simulink model "PlanarRobot5link"  (R2022b)
settings: Solver=VariableStepAuto  StartTime=0.0  StopTime=30  RelTol=1e-3
values from neighbouring files (symbols this model uses):
  I = [1; 1; 1; 0.5; 0.5]*0.2    [RobDyn4link.m]
  l = [1; 1; 1; 1; 2]*0.2    [RobDyn4link.m]
  lc = l./2    [RobDyn4link.m]
  m = [1; 1; 1; 0.3; 0.3]*1    [RobDyn4link.m]
  q0 = [pi/2; -pi/4; -1*pi/6;-pi/12;0;]    [RobDyn4link.m]
  theta_max = [0.915*pi; 0.915*pi; 0.915*pi; 0.915*pi; 0.915*pi;]    [RobDyn4link.m]
  theta_min = [-0.915*pi; -0.915*pi; -0.915*pi; -0.915*pi; -0.915*pi;]    [RobDyn4link.m]
libraries: slpidlib x1
(part 2 of 3)

== matlab function PlanarRobot5link/Subsystem1/MATLAB Function ==
  data: theta input; C output; dtheta input; m input; l input; lc input
function C = fcn(theta,dtheta,m,l,lc)
theta1 = theta(1); theta2 = theta(2); theta3 = theta(3); theta4 = theta(4); theta5 = theta(5);
dtheta1 = dtheta(1); dtheta2 = dtheta(2); dtheta3 = dtheta(3); dtheta4 = dtheta(4); dtheta5 = dtheta(5);
% I1 = I(1); I2 = I(2); I3 = I(3); I4 = I(4); I5 = I(5);
m1 = m(1); m2 = m(2); m3 = m(3); m4 = m(4); m5 = m(5);
l1 = l(1); l2 = l(2); l3 = l(3); l4 = l(4); l5 = l(5);
lc1 = lc(1); lc2 = lc(2); lc3 = lc(3); lc4 = lc(4); lc5 = lc(5);

 
C =[- dtheta2*l1*l4*m5*sin(theta2 + theta3 + theta4) - dtheta3*l1*l4*m5*sin(theta2 + theta3 + theta4) - dtheta4*l1*l4*m5*sin(theta2 + theta3 + theta4) - dtheta2*l1*lc4*m4*sin(theta2 + theta3 + theta4) - dtheta3*l1*lc4*m4*sin(theta2 + theta3 + theta4) - dtheta4*l1*lc4*m4*sin(theta2 + theta3 + theta4) - dtheta3*l2*lc5*m5*sin(theta3 + theta4 + theta5) - dtheta4*l2*lc5*m5*sin(theta3 + theta4 + theta5) - dtheta5*l2*lc5*m5*sin(theta3 + theta4 + theta5) - dtheta2*l1*lc5*m5*sin(theta2 + theta3 + theta4 + theta5) - dtheta3*l1*lc5*m5*sin(theta2 + theta3 + theta4 + theta5) - dtheta4*l1*lc5*m5*sin(theta2 + theta3 + theta4 + theta5) - dtheta5*l1*lc5*m5*sin(theta2 + theta3 + theta4 + theta5) - dtheta2*l1*l3*m4*sin(theta2 + theta3) - dtheta2*l1*l3*m5*sin(theta2 + theta3) - dtheta3*l1*l3*m4*sin(theta2 + theta3) - dtheta3*l1*l3*m5*sin(theta2 + theta3) - dtheta3*l2*l4*m5*sin(theta3 + theta4) - dtheta4*l2*l4*m5*sin(theta3 + theta4) - dtheta2*l1*lc3*m3*sin(theta2 + theta3) - dtheta3*l1*lc3*m3*sin(theta2 + theta3) - dtheta3*l2*lc4*m4*sin(theta3 + theta4) - dtheta4*l2*lc4*m4*sin(theta3 + theta4) - dtheta4*l3*lc5*m5*sin(theta4 + theta5) - dtheta5*l3*lc5*m5*sin(theta4 + theta5) - dtheta2*l1*l2*m3*sin(theta2) - dtheta2*l1*l2*m4*sin(theta2) - dtheta2*l1*l2*m5*sin(theta2) - dtheta3*l2*l3*m4*sin(theta3) - dtheta3*l2*l3*m5*sin(theta3) - dtheta4*l3*l4*m5*sin(theta4) - dtheta2*l1*lc2*m2*sin(theta2) - dtheta3*l2*lc3*m3*sin(theta3) - dtheta4*l3*lc4*m4*sin(theta4) - dtheta5*l4*lc5*m5*sin(theta5), - dtheta1*l1*l4*m5*sin(theta2 + theta3 + theta4) - dtheta2*l1*l4*m5*sin(theta2 + theta3 + theta4) - dtheta3*l1*l4*m5*sin(theta2 + theta3 + theta4) - dtheta4*l1*l4*m5*sin(theta2 + theta3 + theta4) - dtheta1*l1*lc4*m4*sin(theta2 + theta3 + theta4) - dtheta2*l1*lc4*m4*sin(theta2 + theta3 + theta4) - dtheta3*l1*lc4*m4*sin(theta2 + theta3 + theta4) - dtheta4*l1*lc4*m4*sin(theta2 + theta3 + theta4) - dtheta3*l2*lc5*m5*sin(theta3 + theta4 + theta5) - dtheta4*l2*lc5*m5*sin(theta3 + theta4 + theta5) - dtheta5*l2*lc5*m5*sin(theta3 + theta4 + theta5) - dtheta1*l1*lc5*m5*sin(theta2 + theta3 + theta4 + theta5) - dtheta2*l1*lc5*m5*sin(theta2 + theta3 + theta4 + theta5) - dtheta3*l1*lc5*m5*sin(theta2 + theta3 + theta4 + theta5) - dtheta4*l1*lc5*m5*sin(theta2 + theta3 + theta4 + theta5) - dtheta5*l1*lc5*m5*sin(theta2 + theta3 + theta4 + theta5) - dtheta1*l1*l3*m4*sin(theta2 + theta3) - dtheta1*l1*l3*m5*sin(theta2 + theta3) - dtheta2*l1*l3*m4*sin(theta2 + theta3) - dtheta2*l1*l3*m5*sin(theta2 + theta3) - dtheta3*l1*l3*m4*sin(theta2 + theta3) - dtheta3*l1*l3*m5*sin(theta2 + theta3) - dtheta3*l2*l4*m5*sin(theta3 + theta4) - dtheta4*l2*l4*m5*sin(theta3 + theta4) - dtheta1*l1*lc3*m3*sin(theta2 + theta3) - dtheta2*l1*lc3*m3*sin(theta2 + theta3) - dtheta3*l1*lc3*m3*sin(theta2 + theta3) - dtheta3*l2*lc4*m4*sin(theta3 + theta4) - dtheta4*l2*lc4*m4*sin(theta3 + theta4) - dtheta4*l3*lc5*m5*sin(theta4 + theta5) - dtheta5*l3*lc5*m5*sin(theta4 + theta5) - dtheta1*l1*l2*m3*sin(theta2) - dtheta1*l1*l2*m4*sin(theta2) - dtheta2*l1*l2*m3*sin(theta2) - dtheta1*l1*l2*m5*sin(theta2) - dtheta2*l1*l2*m4*sin(theta2) - dtheta2*l1*l2*m5*sin(theta2) - dtheta3*l2*l3*m4*sin(theta3) - dtheta3*l2*l3*m5*sin(theta3) - dtheta4*l3*l4*m5*sin(theta4) - dtheta1*l1*lc2*m2*sin(theta2) - dtheta2*l1*lc2*m2*sin(theta2) - dtheta3*l2*lc3*m3*sin(theta3) - dtheta4*l3*lc4*m4*sin(theta4) - dtheta5*l4*lc5*m5*sin(theta5), - dtheta1*l1*l4*m5*sin(theta2 + theta3 + theta4) - dtheta2*l1*l4*m5*sin(theta2 + theta3 + theta4) - dtheta3*l1*l4*m5*sin(theta2 + theta3 + theta4) - dtheta4*l1*l4*m5*sin(theta2 + theta3 + theta4) - dtheta1*l1*lc4*m4*sin(theta2 + theta3 + theta4) - dtheta2*l1*lc4*m4*sin(theta2 + theta3 + theta4) - dtheta3*l1*lc4*m4*sin(theta2 + theta3 + theta4) - dtheta4*l1*lc4*m4*sin(theta2 + theta3 + theta4) - dtheta1*l2*lc5*m5*sin(theta3 + theta4 + theta5) - dtheta2*l2*lc5*m5*sin(theta3 + theta4 + theta5) - dtheta3*l2*lc5*m5*sin(theta3 + theta4 + theta5) - dtheta4*l2*lc5*m5*sin(theta3 + theta4 + theta5) - dtheta5*l2*lc5*m5*sin(theta3 + theta4 + theta5) - dtheta1*l1*lc5*m5*sin(theta2 + theta3 + theta4 + theta5) - dtheta2*l1*lc5*m5*sin(theta2 + theta3 + theta4 + theta5) - dtheta3*l1*lc5*m5*sin(theta2 + theta3 + theta4 + theta5) - dtheta4*l1*lc5*m5*sin(theta2 + theta3 + theta4 + theta5) - dtheta5*l1*lc5*m5*sin(theta2 + theta3 + theta4 + theta5) - dtheta1*l1*l3*m4*sin(theta2 + theta3) - dtheta1*l1*l3*m5*sin(theta2 + theta3) - dtheta2*l1*l3*m4*sin(theta2 + theta3) - dtheta2*l1*l3*m5*sin(theta2 + theta3) - dtheta3*l1*l3*m4*sin(theta2 + theta3) - dtheta3*l1*l3*m5*sin(theta2 + theta3) - dtheta1*l2*l4*m5*sin(theta3 + theta4) - dtheta2*l2*l4*m5*sin(theta3 + theta4) - dtheta3*l2*l4*m5*sin(theta3 + theta4) - dtheta4*l2*l4*m5*sin(theta3 + theta4) - dtheta1*l1*lc3*m3*sin(theta2 + theta3) - dtheta2*l1*lc3*m3*sin(theta2 + theta3) - dtheta3*l1*lc3*m3*sin(theta2 + theta3) - dtheta1*l2*lc4*m4*sin(theta3 + theta4) - dtheta2*l2*lc4*m4*sin(theta3 + theta4) - dtheta3*l2*lc4*m4*sin(theta3 + theta4) - dtheta4*l2*lc4*m4*sin(theta3 + theta4) - dtheta4*l3*lc5*m5*sin(theta4 + theta5) - dtheta5*l3*lc5*m5*sin(theta4 + theta5) - dtheta1*l2*l3*m4*sin(theta3) - dtheta1*l2*l3*m5*sin(theta3) - dtheta2*l2*l3*m4*sin(theta3) - dtheta2*l2*l3*m5*sin(theta3) - dtheta3*l2*l3*m4*sin(theta3) - dtheta3*l2*l3*m5*sin(theta3) - dtheta4*l3*l4*m5*sin(theta4) - dtheta1*l2*lc3*m3*sin(theta3) - dtheta2*l2*lc3*m3*sin(theta3) - dtheta3*l2*lc3*m3*sin(theta3) - dtheta4*l3*lc4*m4*sin(theta4) - dtheta5*l4*lc5*m5*sin(theta5), - dtheta1*l1*l4*m5*sin(theta2 + theta3 + theta4) - dtheta2*l1*l4*m5*sin(theta2 + theta3 + theta4) - dtheta3*l1*l4*m5*sin(theta2 + theta3 + theta4) - dtheta4*l1*l4*m5*sin(theta2 + theta3 + theta4) - dtheta1*l1*lc4*m4*sin(theta2 + theta3 + theta4) - dtheta2*l1*lc4*m4*sin(theta2 + theta3 + theta4) - dtheta3*l1*lc4*m4*sin(theta2 + theta3 + theta4) - dtheta4*l1*lc4*m4*sin(theta2 + theta3 + theta4) - dtheta1*l2*lc5*m5*sin(theta3 + theta4 + theta5) - dtheta2*l2*lc5*m5*sin(theta3 + theta4 + theta5) - dtheta3*l2*lc5*m5*sin(theta3 + theta4 + theta5) - dtheta4*l2*lc5*m5*sin(theta3 + theta4 + theta5) - dtheta5*l2*lc5*m5*sin(theta3 + theta4 + theta5) - dtheta1*l1*lc5*m5*sin(theta2 + theta3 + theta4 + theta5) - dtheta2*l1*lc5*m5*sin(theta2 + theta3 + theta4 + theta5) - dtheta3*l1*lc5*m5*sin(theta2 + theta3 + theta4 + theta5) - dtheta4*l1*lc5*m5*sin(theta2 + theta3 + theta4 + theta5) - dtheta5*l1*lc5*m5*sin(theta2 + theta3 + theta4 + theta5) - dtheta1*l2*l4*m5*sin(theta3 + theta4) - dtheta2*l2*l4*m5*sin(theta3 + theta4) - dtheta3*l2*l4*m5*sin(theta3 + theta4) - dtheta4*l2*l4*m5*sin(theta3 + theta4) - dtheta1*l2*lc4*m4*sin(theta3 + theta4) - dtheta2*l2*lc4*m4*sin(theta3 + theta4) - dtheta3*l2*lc4*m4*sin(theta3 + theta4) - dtheta4*l2*lc4*m4*sin(theta3 + theta4) - dtheta1*l3*lc5*m5*sin(theta4 + theta5) - dtheta2*l3*lc5*m5*sin(theta4 + theta5) - dtheta3*l3*lc5*m5*sin(theta4 + theta5) - dtheta4*l3*lc5*m5*sin(theta4 + theta5) - dtheta5*l3*lc5*m5*sin(theta4 + theta5) - dtheta1*l3*l4*m5*sin(theta4) - dtheta2*l3*l4*m5*sin(theta4) - dtheta3*l3*l4*m5*sin(theta4) - dtheta4*l3*l4*m5*sin(theta4) - dtheta1*l3*lc4*m4*sin(theta4) - dtheta2*l3*lc4*m4*sin(theta4) - dtheta3*l3*lc4*m4*sin(theta4) - dtheta4*l3*lc4*m4*sin(theta4) - dtheta5*l4*lc5*m5*sin(theta5), -lc5*m5*(l1*sin(theta2 + theta3 + theta4 + theta5) + l3*sin(theta4 + theta5) + l4*sin(theta5) + l2*sin(theta3 + theta4 + theta5))*(dtheta1 + dtheta2 + dtheta3 + dtheta4 + dtheta5);
                                                                                                                                                                                                                                                                                                                                                                                                                                                                                                                  dtheta1*l1*l4*m5*sin(theta2 + theta3 + theta4) + dtheta1*l1*lc4*m4*sin(theta2 + theta3 + theta4) - dtheta3*l2*lc5*m5*sin(theta3 + theta4 + theta5) - dtheta4*l2*lc5*m5*sin(theta3 + theta4 + theta5) - dtheta5*l2*lc5*m5*sin(theta3 + theta4 + theta5) + dtheta1*l1*lc5*m5*sin(theta2 + theta3 + theta4 + theta5) + dtheta1*l1*l3*m4*sin(theta2 + theta3) + dtheta1*l1*l3*m5*sin(theta2 + theta3) - dtheta3*l2*l4*m5*sin(theta3 + theta4) - dtheta4*l2*l4*m5*sin(theta3 + theta4) + dtheta1*l1*lc3*m3*sin(theta2 + theta3) - dtheta3*l2*lc4*m4*sin(theta3 + theta4) - dtheta4*l2*lc4*m4*sin(theta3 + theta4) - dtheta4*l3*lc5*m5*sin(theta4 + theta5) - dtheta5*l3*lc5*m5*sin(theta4 + theta5) + dtheta1*l1*l2*m3*sin(theta2) + dtheta1*l1*l2*m4*sin(theta2) + dtheta1*l1*l2*m5*sin(theta2) - dtheta3*l2*l3*m4*sin(theta3) - dtheta3*l2*l3*m5*sin(theta3) - dtheta4*l3*l4*m5*sin(theta4) + dtheta1*l1*lc2*m2*sin(theta2) - dtheta3*l2*lc3*m3*sin(theta3) - dtheta4*l3*lc4*m4*sin(theta4) - dtheta5*l4*lc5*m5*sin(theta5),                                                                                                                                                                                                                                                                                                                                                                                                                                                                                                                                                                                                                                                                                                                                                                                                                                                                                                                                                                                                                                                                                                                                                                                                                                                                                                                                                                                                                                                                                - dtheta4*(l2*l4*m5*sin(theta3 + theta4) + l2*lc4*m4*sin(theta3 + theta4) + l3*lc5*m5*sin(theta4 + theta5) + l3*l4*m5*sin(theta4) + l3*lc4*m4*sin(theta4) + l2*lc5*m5*sin(theta3 + theta4 + theta5)) - dtheta3*l2*(l3*m4*sin(theta3) + l3*m5*sin(theta3) + lc3*m3*sin(theta3) + lc5*m5*sin(theta3 + theta4 + theta5) + l4*m5*sin(theta3 + theta4) + lc4*m4*sin(theta3 + theta4)) - dtheta5*lc5*m5*(l3*sin(theta4 + theta5) + l4*sin(theta5) + l2*sin(theta3 + theta4 + theta5)),                                                                                                                                                                                                                                                                                                                                                                                                                                                                                                                                                                                                                                                                                                                                                                                                                                                                                                                                                                                                                                                                                               - dtheta1*l2*lc5*m5*sin(theta3 + theta4 + theta5) - dtheta2*l2*lc5*m5*sin(theta3 + theta4 + theta5) - dtheta3*l2*lc5*m5*sin(theta3 + theta4 + theta5) - dtheta4*l2*lc5*m5*sin(theta3 + theta4 + theta5) - dtheta5*l2*lc5*m5*sin(theta3 + theta4 + theta5) - dtheta1*l2*l4*m5*sin(theta3 + theta4) - dtheta2*l2*l4*m5*sin(theta3 + theta4) - dtheta3*l2*l4*m5*sin(theta3 + theta4) - dtheta4*l2*l4*m5*sin(theta3 + theta4) - dtheta1*l2*lc4*m4*sin(theta3 + theta4) - dtheta2*l2*lc4*m4*sin(theta3 + theta4) - dtheta3*l2*lc4*m4*sin(theta3 + theta4) - dtheta4*l2*lc4*m4*sin(theta3 + theta4) - dtheta4*l3*lc5*m5*sin(theta4 + theta5) - dtheta5*l3*lc5*m5*sin(theta4 + theta5) - dtheta1*l2*l3*m4*sin(theta3) - dtheta1*l2*l3*m5*sin(theta3) - dtheta2*l2*l3*m4*sin(theta3) - dtheta2*l2*l3*m5*sin(theta3) - dtheta3*l2*l3*m4*sin(theta3) - dtheta3*l2*l3*m5*sin(theta3) - dtheta4*l3*l4*m5*sin(theta4) - dtheta1*l2*lc3*m3*sin(theta3) - dtheta2*l2*lc3*m3*sin(theta3) - dtheta3*l2*lc3*m3*sin(theta3) - dtheta4*l3*lc4*m4*sin(theta4) - dtheta5*l4*lc5*m5*sin(theta5),                                                                                                                                                                                                                                                                                                                                                                                                                                                                                                                                                                                                                                                                                                                    - dtheta1*l2*lc5*m5*sin(theta3 + theta4 + theta5) - dtheta2*l2*lc5*m5*sin(theta3 + theta4 + theta5) - dtheta3*l2*lc5*m5*sin(theta3 + theta4 + theta5) - dtheta4*l2*lc5*m5*sin(theta3 + theta4 + theta5) - dtheta5*l2*lc5*m5*sin(theta3 + theta4 + theta5) - dtheta1*l2*l4*m5*sin(theta3 + theta4) - dtheta2*l2*l4*m5*sin(theta3 + theta4) - dtheta3*l2*l4*m5*sin(theta3 + theta4) - dtheta4*l2*l4*m5*sin(theta3 + theta4) - dtheta1*l2*lc4*m4*sin(theta3 + theta4) - dtheta2*l2*lc4*m4*sin(theta3 + theta4) - dtheta3*l2*lc4*m4*sin(theta3 + theta4) - dtheta4*l2*lc4*m4*sin(theta3 + theta4) - dtheta1*l3*lc5*m5*sin(theta4 + theta5) - dtheta2*l3*lc5*m5*sin(theta4 + theta5) - dtheta3*l3*lc5*m5*sin(theta4 + theta5) - dtheta4*l3*lc5*m5*sin(theta4 + theta5) - dtheta5*l3*lc5*m5*sin(theta4 + theta5) - dtheta1*l3*l4*m5*sin(theta4) - dtheta2*l3*l4*m5*sin(theta4) - dtheta3*l3*l4*m5*sin(theta4) - dtheta4*l3*l4*m5*sin(theta4) - dtheta1*l3*lc4*m4*sin(theta4) - dtheta2*l3*lc4*m4*sin(theta4) - dtheta3*l3*lc4*m4*sin(theta4) - dtheta4*l3*lc4*m4*sin(theta4) - dtheta5*l4*lc5*m5*sin(theta5),                                             -lc5*m5*(l3*sin(theta4 + theta5) + l4*sin(theta5) + l2*sin(theta3 + theta4 + theta5))*(dtheta1 + dtheta2 + dtheta3 + dtheta4 + dtheta5);
                                                                                                                                                                                                                                                                                                                                                                                                                                                                                                                                                                                                   dtheta1*l1*l4*m5*sin(theta2 + theta3 + theta4) + dtheta1*l1*lc4*m4*sin(theta2 + theta3 + theta4) + dtheta1*l2*lc5*m5*sin(theta3 + theta4 + theta5) + dtheta2*l2*lc5*m5*sin(theta3 + theta4 + theta5) + dtheta1*l1*lc5*m5*sin(theta2 + theta3 + theta4 + theta5) + dtheta1*l1*l3*m4*sin(theta2 + theta3) + dtheta1*l1*l3*m5*sin(theta2 + theta3) + dtheta1*l2*l4*m5*sin(theta3 + theta4) + dtheta2*l2*l4*m5*sin(theta3 + theta4) + dtheta1*l1*lc3*m3*sin(theta2 + theta3) + dtheta1*l2*lc4*m4*sin(theta3 + theta4) + dtheta2*l2*lc4*m4*sin(theta3 + theta4) - dtheta4*l3*lc5*m5*sin(theta4 + theta5) - dtheta5*l3*lc5*m5*sin(theta4 + theta5) + dtheta1*l2*l3*m4*sin(theta3) + dtheta1*l2*l3*m5*sin(theta3) + dtheta2*l2*l3*m4*sin(theta3) + dtheta2*l2*l3*m5*sin(theta3) - dtheta4*l3*l4*m5*sin(theta4) + dtheta1*l2*lc3*m3*sin(theta3) + dtheta2*l2*lc3*m3*sin(theta3) - dtheta4*l3*lc4*m4*sin(theta4) - dtheta5*l4*lc5*m5*sin(theta5),                                                                                                                                                                                                                                                                                                                                                                                                                                                                                                                                                                                                                                                                                                                                                                                                                                                                                                                                                                                                                                                                                                                                                                                                                                                                                                                                                                                                               dtheta1*(l2*l4*m5*sin(theta3 + theta4) + l2*lc4*m4*sin(theta3 + theta4) + l2*l3*m4*sin(theta3) + l2*l3*m5*sin(theta3) + l2*lc3*m3*sin(theta3) + l2*lc5*m5*sin(theta3 + theta4 + theta5)) - dtheta5*(l3*lc5*m5*sin(theta4 + theta5) + l4*lc5*m5*sin(theta5)) + dtheta2*(l2*l4*m5*sin(theta3 + theta4) + l2*lc4*m4*sin(theta3 + theta4) + l2*l3*m4*sin(theta3) + l2*l3*m5*sin(theta3) + l2*lc3*m3*sin(theta3) + l2*lc5*m5*sin(theta3 + theta4 + theta5)) - dtheta4*(l3*lc5*m5*sin(theta4 + theta5) + l3*l4*m5*sin(theta4) + l3*lc4*m4*sin(theta4)),                                                                                                                                                                                                                                                                                                                                                                                                                                                                                                                                                                                                                                                                                                                                                                                                                                                                                                                                                                                                                                                                                                                                                                                                                                                                                                                                                                                                                                                                                                                                                                                                                                                                                                                                                                                                                                                                                                                                                                                                           - dtheta5*(l3*lc5*m5*sin(theta4 + theta5) + l4*lc5*m5*sin(theta5)) - dtheta4*(l3*lc5*m5*sin(theta4 + theta5) + l3*l4*m5*sin(theta4) + l3*lc4*m4*sin(theta4)),                                                                                                                                                                                                                                                                                                                                                                                                                                                                                                                                                                                                                                                                                                                                                                                                                                                                                                                                                                                                                                                                                                                                                                                                                                                                                                                                                                                                               - dtheta1*l3*(l4*m5*sin(theta4) + lc4*m4*sin(theta4) + lc5*m5*sin(theta4 + theta5)) - dtheta2*l3*(l4*m5*sin(theta4) + lc4*m4*sin(theta4) + lc5*m5*sin(theta4 + theta5)) - dtheta3*l3*(l4*m5*sin(theta4) + lc4*m4*sin(theta4) + lc5*m5*sin(theta4 + theta5)) - dtheta4*l3*(l4*m5*sin(theta4) + lc4*m4*sin(theta4) + lc5*m5*sin(theta4 + theta5)) - dtheta5*lc5*m5*(l3*sin(theta4 + theta5) + l4*sin(theta5)),                                                                                -lc5*m5*(l3*sin(theta4 + theta5) + l4*sin(theta5))*(dtheta1 + dtheta2 + dtheta3 + dtheta4 + dtheta5);
                                                                                                                                                                                                                                                                                                                                                                                                                                                                                                                                                                                                                                                                                                                                                 dtheta1*l1*l4*m5*sin(theta2 + theta3 + theta4) + dtheta1*l1*lc4*m4*sin(theta2 + theta3 + theta4) + dtheta1*l2*lc5*m5*sin(theta3 + theta4 + theta5) + dtheta2*l2*lc5*m5*sin(theta3 + theta4 + theta5) + dtheta1*l1*lc5*m5*sin(theta2 + theta3 + theta4 + theta5) + dtheta1*l2*l4*m5*sin(theta3 + theta4) + dtheta2*l2*l4*m5*sin(theta3 + theta4) + dtheta1*l2*lc4*m4*sin(theta3 + theta4) + dtheta2*l2*lc4*m4*sin(theta3 + theta4) + dtheta1*l3*lc5*m5*sin(theta4 + theta5) + dtheta2*l3*lc5*m5*sin(theta4 + theta5) + dtheta3*l3*lc5*m5*sin(theta4 + theta5) + dtheta1*l3*l4*m5*sin(theta4) + dtheta2*l3*l4*m5*sin(theta4) + dtheta3*l3*l4*m5*sin(theta4) + dtheta1*l3*lc4*m4*sin(theta4) + dtheta2*l3*lc4*m4*sin(theta4) + dtheta3*l3*lc4*m4*sin(theta4) - dtheta5*l4*lc5*m5*sin(theta5),                                                                                                                                                                                                                                                                                                                                                                                                                                                                                                                                                                                                                                                                                                                                                                                                                                                                                                                                                                                                                                                                                                                                                                                                                                                                                                                                    dtheta1*l2*lc5*m5*sin(theta3 + theta4 + theta5) + dtheta2*l2*lc5*m5*sin(theta3 + theta4 + theta5) + dtheta1*l2*l4*m5*sin(theta3 + theta4) + dtheta2*l2*l4*m5*sin(theta3 + theta4) + dtheta1*l2*lc4*m4*sin(theta3 + theta4) + dtheta2*l2*lc4*m4*sin(theta3 + theta4) + dtheta1*l3*lc5*m5*sin(theta4 + theta5) + dtheta2*l3*lc5*m5*sin(theta4 + theta5) + dtheta3*l3*lc5*m5*sin(theta4 + theta5) + dtheta1*l3*l4*m5*sin(theta4) + dtheta2*l3*l4*m5*sin(theta4) + dtheta3*l3*l4*m5*sin(theta4) + dtheta1*l3*lc4*m4*sin(theta4) + dtheta2*l3*lc4*m4*sin(theta4) + dtheta3*l3*lc4*m4*sin(theta4) - dtheta5*l4*lc5*m5*sin(theta5),                                                                                                                                                                                                                                                                                                                                                                                                                                                                                                                                                                                                                                                                                                                                                                                                                                                                                                                                                                                                                                                                                                                                                                                                                                                                                                                                                                                                                                                                                                                                                                                                                                                                                                                                                                                                                                                                              dtheta1*l3*(l4*m5*sin(theta4) + lc4*m4*sin(theta4) + lc5*m5*sin(theta4 + theta5)) + dtheta2*l3*(l4*m5*sin(theta4) + lc4*m4*sin(theta4) + lc5*m5*sin(theta4 + theta5)) + dtheta3*l3*(l4*m5*sin(theta4) + lc4*m4*sin(theta4) + lc5*m5*sin(theta4 + theta5)) - dtheta5*l4*lc5*m5*sin(theta5),                                                                                                                                                                                                                                                                                                                                                                                                                                                                                                                                                                                                                                                                                                                                                                                                                                                                                                                                                                                                                                                                                                                                                                                                                                                                                                                                                                                                                                                                                                                                                                                                                                                                                                                                                                                            -dtheta5*l4*lc5*m5*sin(theta5),                                                                                                            -l4*lc5*m5*sin(theta5)*(dtheta1 + dtheta2 + dtheta3 + dtheta4 + dtheta5);
                                                                                                                                                                                                                                                                                                                                                                                                                                                                                                                                                                                                                                                                                                                                                                                                                                                                                                                                                                                                                                                                                                                                                                                lc5*m5*(dtheta1*l4*sin(theta5) + dtheta2*l4*sin(theta5) + dtheta3*l4*sin(theta5) + dtheta4*l4*sin(theta5) + dtheta1*l2*sin(theta3 + theta4 + theta5) + dtheta2*l2*sin(theta3 + theta4 + theta5) + dtheta1*l1*sin(theta2 + theta3 + theta4 + theta5) + dtheta1*l3*sin(theta4 + theta5) + dtheta2*l3*sin(theta4 + theta5) + dtheta3*l3*sin(theta4 + theta5)),                                                                                                                                                                                                                                                                                                                                                                                                                                                                                                                                                                                                                                                                                                                                                                                                                                                                                                                                                                                                                                                                                                                                                                                                                                                                                                                                                                                                                                                                                                                                                                                                                                                         lc5*m5*(dtheta1*l4*sin(theta5) + dtheta2*l4*sin(theta5) + dtheta3*l4*sin(theta5) + dtheta4*l4*sin(theta5) + dtheta1*l2*sin(theta3 + theta4 + theta5) + dtheta2*l2*sin(theta3 + theta4 + theta5) + dtheta1*l3*sin(theta4 + theta5) + dtheta2*l3*sin(theta4 + theta5) + dtheta3*l3*sin(theta4 + theta5)),                                                                                                                                                                                                                                                                                                                                                                                                                                                                                                                                                                                                                                                                                                                                                                                                                                                                                                                                                                                                                                                                                                                                                                                                                                                                                                                                                                                                                                                                                                                                                                                                                                                                                                                                                                                                                                                                                                                                                       lc5*m5*(dtheta1*l4*sin(theta5) + dtheta2*l4*sin(theta5) + dtheta3*l4*sin(theta5) + dtheta4*l4*sin(theta5) + dtheta1*l3*sin(theta4 + theta5) + dtheta2*l3*sin(theta4 + theta5) + dtheta3*l3*sin(theta4 + theta5)),                                                                                                                                                                                                                                                                                                                                                                                                                                                                                                                                                                                                                                                                                                                                                                                                                                                                                                                                                                                                                                                                                                                                                                                                                                                                                                                                                                                                                                                                                                                                                                                                                                                                                                                                                             l4*lc5*m5*sin(theta5)*(dtheta1 + dtheta2 + dtheta3 + dtheta4),                                                                                                                                                                                   0;];

== matlab function PlanarRobot5link/Subsystem6/MATLAB Function1 ==
  data: Jc output; Jc_pinv output; J_general input; P output; Jee input; M input; Pnull output; Mc output; Lambda_c output
function [Jc,Jc_pinv,P,Pnull,Mc,Lambda_c] = fcn(J_general,Jee,M)
Jc = J_general(2:3,:);
% JcJcinv = (Jc*Jc')\eye(2);
Jc_pinv = Jc'/(Jc*Jc');
P = Jc_pinv*Jc;
Pnull = eye(5) - P;
Mc = P*M + eye(5) - P;
Lambda_c = (Jee * (Mc \ P) * Jee' + 1e-3*eye(3)) \ eye(3);

== matlab function PlanarRobot5link/Subsystem6/MATLAB Function2 ==
  data: C input; Jc_dot input; Jc_pinv input; hc output; P input; Lambda_c input; Jee input; Jeedot input; thetadot input; Mc input
function hc = fcn(C,Jc_dot,Jc_pinv,P,Lambda_c,Jee,Jeedot,thetadot,Mc)
Pdot = -Jc_pinv*Jc_dot*P - P*Jc_dot'*Jc_pinv';
hc = Lambda_c*Jee/Mc*(P*C*thetadot - Pdot*thetadot)-Lambda_c*Jeedot*thetadot;

== matlab function PlanarRobot5link/Subsystem6/MATLAB Function3 ==
  data: Lambda_c_dot input; pdot_r0 output; tau input; hc input; Jee input; xdot input; r input
function pdot_r0 = fcn(Lambda_c_dot,tau,hc,Jee,xdot,r)
Jee_pinv = Jee'/(Jee*Jee');
F = Jee_pinv'*tau;
pdot_r0 = Lambda_c_dot*xdot + F - hc + r;
